simulink model "Block_fixedQ_Ccode_ideal"  (R2017b)
settings: Solver=ode45  StartTime=0.0  StopTime=Test_time  RelTol=1e-3
values from neighbouring files (symbols this model uses):
  Lq = length(F.Omega(:,:,1))    [Saveconstraints.m]
  Ts = plant.Ts    [CoprimeFactorizationSS.m]    (also in ID_Model.m = 0.001; ID_Model_4.m = 0.001; ID_Model_ITRI.m = 0.001; gConstraintFun.m = P.Ts)
undefined symbols (not defined in the file or in its folder): ccA, ccB, ccC, ccD, plant
settings Model: Creator=LAB_JHU  LastModifiedBy=LAB_JHU
settings DataIOCC: LimitDataPoints=on  SaveFormat=Array  SignalLoggingSaveFormat=ModelDataLogs
settings OptimizationCC: BlockReduction=off  BooleanDataType=off  LifeSpan=inf
settings DebuggingCC: SaveWithParameterizedLinksMsg=none  UnderspecifiedInitializationDetection=Classic  MergeDetectMultiDrivingBlocksExec=none  SignalResolutionControl=TryResolveAllWithWarning  MultiTaskDSMMsg=warning  MultiTaskCondExecSysMsg=none  StateNameClashWarn=warning  StrictBusMsg=None  SFUnexpectedBacktrackingDiag=warning  SFNoUnconditionalDefaultTransitionDiag=warning  SFExecutionAtInitializationDiag=none
settings HardwareCC: ProdBitPerPointer=32  ProdBitPerSizeT=32  ProdBitPerPtrDiffT=32  ProdLargestAtomicFloat=None  ProdIntDivRoundTo=Undefined  ProdEndianess=Unspecified  ProdWordSize=32  ProdHWDeviceType=32-bit Generic  TargetUnknown=on
settings ModelReferenceCC: PropagateSignalLabelsOutOfModel=off
settings CodeAppCC: StateflowObjectComments=on
settings GRTTargetCC: TargetLangStandard=C89/C90 (ANSI)  GeneratePreprocessorConditionals=Disable all
settings ConfigComp: CovMetricSettings=dw  CovHtmlReporting=on  CovSaveCumulativeToWorkspaceVar=on  CovSaveSingleToWorkspaceVar=on  CovExternalEMLEnable=off

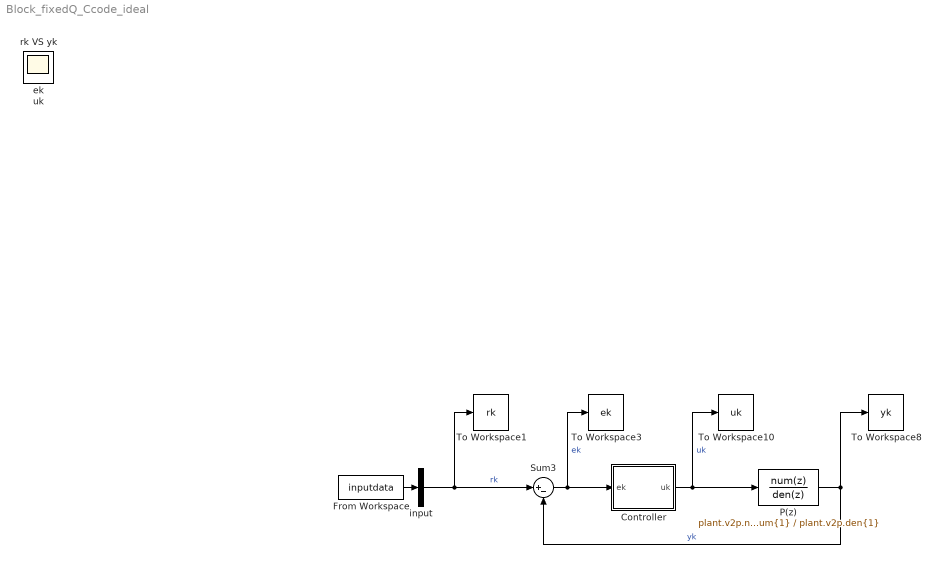
== system Block_fixedQ_Ccode_ideal ==
  Controller : Subsystem
  From Workspace : FromWorkspace  VariableName=inputdata  SampleTime=Ts
  P(z) : DiscreteTransferFcn  Numerator=plant.v2p.num{1}  Denominator=plant.v2p.den{1}  SampleTime=Ts
  Sum3 : Sum  Inputs=|+-
  To Workspace1 : ToWorkspace  VariableName=rk  SampleTime=-1
  To Workspace10 : ToWorkspace  VariableName=uk  SampleTime=-1
  To Workspace3 : ToWorkspace  VariableName=ek  SampleTime=-1
  To Workspace8 : ToWorkspace  VariableName=yk  SampleTime=-1
  input : Demux  Outputs=1
  ek : Scope
  rk VS yk : Scope
  uk : Scope
  wires:
  input/1 -> Sum3/1, To Workspace1/1  "rk"
  P(z)/1 -> Sum3/2, To Workspace8/1  "yk"
  Sum3/1 -> Controller/1(ek), To Workspace3/1  "ek"
  Controller/1(uk) -> P(z)/1, To Workspace10/1  "uk"
  From Workspace/1 -> input/1

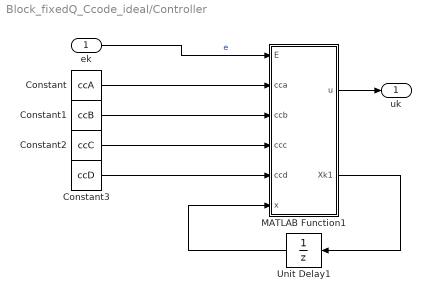
== system Block_fixedQ_Ccode_ideal/Controller ==
  ek : Inport
  Constant : Constant  Value=ccA  VectorParams1D=off
  Constant1 : Constant  Value=ccB  VectorParams1D=off
  Constant2 : Constant  Value=ccC  VectorParams1D=off
  Constant3 : Constant  Value=ccD  VectorParams1D=off
  MATLAB Function1 : MATLAB Function  TreatAsAtomicUnit=on
  Unit Delay1 : UnitDelay  InitialCondition=zeros(Lq+4,1)  SampleTime=-1
  uk : Outport
  wires:
  Unit Delay1/1 -> MATLAB Function1/6(x)
  MATLAB Function1/2(Xk1) -> Unit Delay1/1
  Constant/1 -> MATLAB Function1/2(cca)
  Constant1/1 -> MATLAB Function1/3(ccb)
  Constant3/1 -> MATLAB Function1/5(ccd)
  Constant2/1 -> MATLAB Function1/4(ccc)
  ek/1 -> MATLAB Function1/1(E)  "e"
  MATLAB Function1/1(u) -> uk/1

== matlab function Block_fixedQ_Ccode_ideal/Controller/MATLAB Function1 ==
  data: E input; cca input; ccb input; ccc input; ccd input; u output; x input; Xk1 output
function [u,Xk1] = C_Z(E,cca,ccb,ccc,ccd,x)

    Xk1 = cca*x+ccb*E;
    u = ccc*x+ccd*E;
end
